simulink model "TestPLCCoder"  (R2018b)
settings: Solver=FixedStepAuto  StartTime=0.0  StopTime=10.0  FixedStep=0.1  RelTol=1e-3
undefined symbols (not defined in the file): s
libraries: cstblocks x1
settings Model: Creator=Trips  LastModifiedBy=Trips
settings ConfigComp: PLC_TargetIDE=step7  PLC_GenerateReport=off  PLC_LaunchReport=off

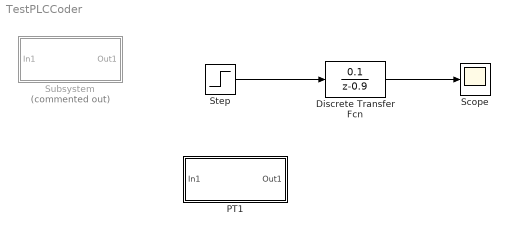
== system TestPLCCoder ==
  Discrete Transfer Fcn : DiscreteTransferFcn  Numerator=[0.1]  Denominator=[1 -0.9]
  PT1 : Subsystem  TreatAsAtomicUnit=on
  Scope : Scope
  Step : Step  SampleTime=0
  Subsystem : Subsystem  Commented=on  TreatAsAtomicUnit=on
  wires:
  Step/1 -> Discrete Transfer Fcn/1
  Discrete Transfer Fcn/1 -> Scope/1

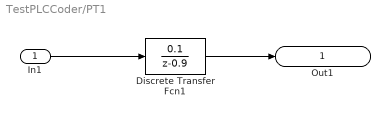
== system TestPLCCoder/PT1 ==
  In1 : Inport
  Discrete Transfer Fcn1 : DiscreteTransferFcn  Numerator=[0.1]  Denominator=[1 -0.9]
  Out1 : Outport
  wires:
  In1/1 -> Discrete Transfer Fcn1/1
  Discrete Transfer Fcn1/1 -> Out1/1

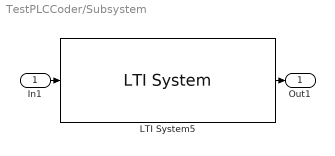
== system TestPLCCoder/Subsystem ==
  In1 : Inport
  LTI System5 : cstblocks/LTI System  sys=1.75/(3107*s+1)*exp(-206*s)  IC=[]
  Out1 : Outport
  wires:
  In1/1 -> LTI System5/1
  LTI System5/1 -> Out1/1
